simulink model "Switch"  (R2024b)
settings: Solver=VariableStepAuto  StartTime=0.0  StopTime=1  FixedStep=50e-6  MaxStep=0.001  MinStep=1e-8
model workspace (MAT data in the model file):
  condition = Simulink.Parameter
  condition.Complexity = 'real'
  condition.Dimensions = [0 0]
  condition.DataType = 'auto'
undefined symbols (not defined in the file or in its folder): DiscIntNeverNeededParam, ee_sli_rtmsupport, gcbh
libraries: spsIdealSwitchLib x12, spsCurrentMeasurementLib x6, spsSeriesRLCBranchLib x6, eeGeneralControl x6, spsControlledVoltageSourceLib x6, spsVoltageMeasurementLib x6, simulink x3, spsAsynchronousMachineSIUnitsLib x2, spsGroundLib x2, spsThreePhaseTransformerInductanceMatrixTypeTwoWindingsLib x1, spspowerguiLib x1
(part 1 of 2)
settings Model: Creator=rishikeshtiwari  LastModifiedBy=Milan Mavani
settings DebuggingCC: IgnoredZcDiagnostic=none

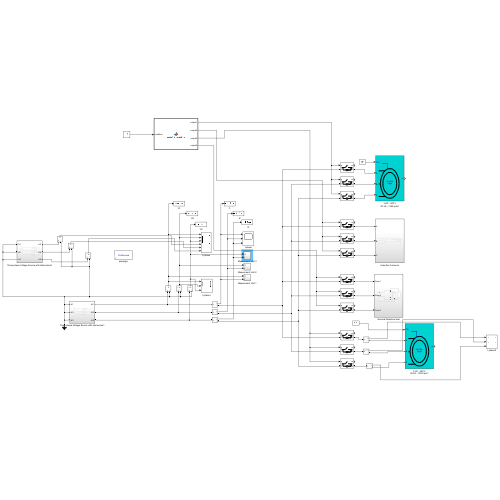
[thumbnail: Simulink's stored preview of the top-level diagram]
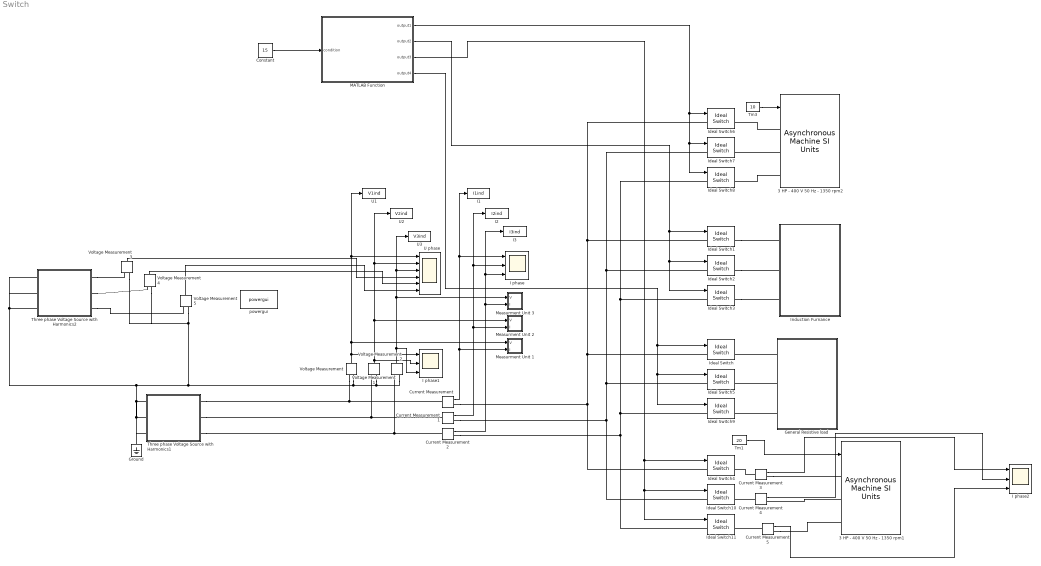
== system Switch ==
  "    I2" : ToWorkspace  VariableName=I2ind  SaveFormat=Timeseries  SampleTime=0.001
  "    I3" : ToWorkspace  VariableName=I3ind  SaveFormat=Timeseries  SampleTime=0.001
  3 HP - 400 V 50 Hz - 1350 rpm1 : spsAsynchronousMachineSIUnitsLib/Asynchronous Machine SI Units  RotorType=Double squirrel-cage  PresetModel=No  MechanicalLoad=Torque Tm  ShowDetailedParameters=on  ReferenceFrame=Stationary  Units=SI  MeasurementBus=on  NominalParameters=[2985 400 50]  VoltageRatio=1  Stator=[3.244 0.00018]  Rotor="[ 0.816  2.0e-3 ]"  Cage1=[1.701 0.01278]  Cage2=[2.063 0.00018]  Lm=0.008931  Mechanical=[0.089 0 1]  PolePairs=2  InitialConditions="[ 1,0   0,0,0   0,0,0 ]"  SimulateSaturation=off  Saturation=[14.03593122, 27.81365428, 53.79336849, 72.68890987, 97.98006896, 148.6815601, 215.7428561, 302.9841135, 428.7778367 ; 230, 322, 414, 460, 506, 552, 598, 644, 690]  LoadFlowParameters=0  TsPowergui=0  TsBlock=-1  IterativeModel=Trapezoidal non iterative  IterativeDiscreteModel=Trapezoidal non iterative  Pmec=0
      settings: AttributesFormatString=\n
  3 HP - 400 V 50 Hz - 1350 rpm2 : spsAsynchronousMachineSIUnitsLib/Asynchronous Machine SI Units  RotorType=Double squirrel-cage  PresetModel=No  MechanicalLoad=Torque Tm  ShowDetailedParameters=on  ReferenceFrame=Stationary  Units=SI  MeasurementBus=on  NominalParameters=[1720.1 400 50]  VoltageRatio=1  Stator=[76.66 0.08155]  Rotor="[ 0.816  2.0e-3 ]"  Cage1=[87.17 0.08486]  Cage2=[87.63 0.08155]  Lm=0.8867  Mechanical=[0.089 0 2]  PolePairs=2  InitialConditions="[ 1,0   0,0,0   0,0,0 ]"  SimulateSaturation=off  Saturation=[14.03593122, 27.81365428, 53.79336849, 72.68890987, 97.98006896, 148.6815601, 215.7428561, 302.9841135, 428.7778367 ; 230, 322, 414, 460, 506, 552, 598, 644, 690]  LoadFlowParameters=0  TsPowergui=0  TsBlock=-1  IterativeModel=Trapezoidal non iterative  IterativeDiscreteModel=Trapezoidal non iterative  Pmec=0
      settings: AttributesFormatString=\n
  Constant : Constant  Value=15  VectorParams1D=off  OutDataTypeStr=Inherit: Inherit via back propagation
  Current Measurement{,1..5} (6 alike) : spsCurrentMeasurementLib/Current Measurement  PhasorSimulation=off  OutputType=Complex  PSBequivalent=0
  General Resistive load : Subsystem
  Ground : spsGroundLib/Ground  LConnTagsString=a
  I phase : Scope  NumInputPorts=3
  I phase1 : Scope  NumInputPorts=3
  I phase2 : Scope  NumInputPorts=3
  I1 : ToWorkspace  VariableName=I1ind  SaveFormat=Timeseries  SampleTime=0.001
  Ideal Switch{,1..11} (12 alike) : spsIdealSwitchLib/Ideal Switch  Ron=0.001  Lon=0  IC=0  Rs=1e10  Cs=inf  Measurements=on
  Induction Furnance : Subsystem
  MATLAB Function : MATLAB Function  TreatAsAtomicUnit=on
  Measurment Unit 1 : Subsystem
  Measurment Unit 2 : Subsystem
  Measurment Unit 3 : Subsystem
  Three phase Voltage Source with Harmonics1 : Subsystem
  Three phase Voltage Source with Harmonics2 : Subsystem
  Tm1 : Constant  Value=20
  Tm3 : Constant  Value=10
  U phase : Scope  NumInputPorts=6
  U1 : ToWorkspace  VariableName=V1ind  SaveFormat=Timeseries  SampleTime=0.001
  U2 : ToWorkspace  VariableName=V2ind  SaveFormat=Timeseries  SampleTime=0.001
  U3 : ToWorkspace  VariableName=V3ind  SaveFormat=Timeseries  SampleTime=0.001
  Voltage Measurement{,1..5} (6 alike) : spsVoltageMeasurementLib/Voltage Measurement  PhasorSimulation=off  OutputType=Complex  PSBequivalent=0
  powergui : spspowerguiLib/powergui  Priority=1  SimulationMode=Continuous  SampleTime=50e-6  frequency=60  Iterations=50  frequencyindice=50  Pbase=100e6  ErrMax=1e-4  UnitsV=kV  UnitsW=MW  buscounter=0  FunctionMessages=off  echomessages=off  EnableUseOfTLC=off  CurrentSourceSwitches=off  DisableSnubberDevices=off  DisableRonSwitches=off  DisableVfSwitches=off  DisplayEquations=off  AutomaticDiscreteSolvers=off  SolverType=Tustin/Backward Euler (TBE)  Interpol=off  ExternalGateDelay=off  methode=off  Ts=100  x0status=blocks  SPID=on  SwTol=0  HookPort=off  NonlinearTolerance=1e-4  nMaxIteration=100  ContinueOnMaxIteration=off  RestoreLinks=warning  ResistiveCurrentMeasurement=off  Frange=[0:2:500]  Ylog=off  Xlog=on  ShowGrid=off  save=off  variable=ZData  structure=0  ZoomFFT=off  StartTime=0.0  cycles=1  DisplayStyle=1  fundamental=60  FreqAxis=off  MaxFrequency=1000  frequencyindicesteady=1  RmsSteady=1  display=off
  wires:
  Tm3/1 -> 3 HP - 400 V 50 Hz - 1350 rpm2/1
  Current Measurement/1 -> Measurment Unit 1/2(I), I1/1, I phase/1
  Current Measurement1/1 -> "    I2"/1, I phase/2, Measurment Unit 2/2(I)
  Current Measurement2/1 -> "    I3"/1, I phase/3, Measurment Unit 3/2(I)
  Voltage Measurement1/1 -> I phase1/2, U2/1, U phase/2, Measurment Unit 2/1(V)
  Voltage Measurement/1 -> I phase1/1, Measurment Unit 1/1(V), U1/1, U phase/1
  MATLAB Function/2(output2) -> Ideal Switch3/1, Ideal Switch2/1, Ideal Switch1/1
  Constant/1 -> MATLAB Function/1(condition)
  MATLAB Function/4(output4) -> Ideal Switch/1, Ideal Switch5/1, Ideal Switch9/1
  MATLAB Function/3(output3) -> Ideal Switch4/1, Ideal Switch10/1, Ideal Switch11/1
  Voltage Measurement3/1 -> U phase/4
  Voltage Measurement4/1 -> U phase/5
  Voltage Measurement5/1 -> U phase/6
  MATLAB Function/1(output1) -> Ideal Switch8/1, Ideal Switch7/1, Ideal Switch6/1
  Tm1/1 -> 3 HP - 400 V 50 Hz - 1350 rpm1/1
  Voltage Measurement2/1 -> U3/1, U phase/3, Measurment Unit 3/1(V), I phase1/3
  Current Measurement3/1 -> I phase2/1
  Current Measurement4/1 -> I phase2/2
  Current Measurement5/1 -> I phase2/3
  connections:
  3 HP - 400 V 50 Hz - 1350 rpm2/LConn2 -- Ideal Switch7/RConn1
  3 HP - 400 V 50 Hz - 1350 rpm2/LConn3 -- Ideal Switch8/RConn1
  3 HP - 400 V 50 Hz - 1350 rpm2/LConn1 -- Ideal Switch6/RConn1
  Voltage Measurement/LConn1 -- Three phase Voltage Source with Harmonics1/RConn1 -- Current Measurement/LConn1
  Voltage Measurement1/LConn2 -- Voltage Measurement2/LConn2 -- Three phase Voltage Source with Harmonics1/LConn1 -- Three phase Voltage Source with Harmonics1/LConn2 -- Three phase Voltage Source with Harmonics1/LConn3 -- Ground/LConn1 -- Three phase Voltage Source with Harmonics2/LConn3 -- Three phase Voltage Source with Harmonics2/LConn2 -- Three phase Voltage Source with Harmonics2/LConn1 -- Voltage Measurement3/LConn2 -- Voltage Measurement4/LConn2 -- Voltage Measurement5/LConn2 -- Voltage Measurement/LConn2
  Current Measurement2/LConn1 -- Three phase Voltage Source with Harmonics1/RConn3 -- Voltage Measurement2/LConn1
  Current Measurement1/LConn1 -- Three phase Voltage Source with Harmonics1/RConn2 -- Voltage Measurement1/LConn1
  Current Measurement/RConn1 -- Ideal Switch/LConn1 -- Ideal Switch6/LConn1 -- Ideal Switch1/LConn1 -- Ideal Switch4/LConn1
  Current Measurement1/RConn1 -- Ideal Switch2/LConn1 -- Ideal Switch7/LConn1 -- Ideal Switch5/LConn1 -- Ideal Switch10/LConn1
  Current Measurement2/RConn1 -- Ideal Switch9/LConn1 -- Ideal Switch3/LConn1 -- Ideal Switch8/LConn1 -- Ideal Switch11/LConn1
  General Resistive load/LConn1 -- Ideal Switch/RConn1
  General Resistive load/LConn2 -- Ideal Switch5/RConn1
  General Resistive load/LConn3 -- Ideal Switch9/RConn1
  Ideal Switch1/RConn1 -- Induction Furnance/LConn1
  Ideal Switch2/RConn1 -- Induction Furnance/LConn2
  Ideal Switch3/RConn1 -- Induction Furnance/LConn3
  Three phase Voltage Source with Harmonics2/RConn1 -- Voltage Measurement3/LConn1
  Three phase Voltage Source with Harmonics2/RConn2 -- Voltage Measurement4/LConn1
  Three phase Voltage Source with Harmonics2/RConn3 -- Voltage Measurement5/LConn1
  Current Measurement5/LConn1 -- Ideal Switch11/RConn1
  Current Measurement4/LConn1 -- Ideal Switch10/RConn1
  Current Measurement3/LConn1 -- Ideal Switch4/RConn1
  Current Measurement3/RConn1 -- 3 HP - 400 V 50 Hz - 1350 rpm1/LConn1
  3 HP - 400 V 50 Hz - 1350 rpm1/LConn2 -- Current Measurement4/RConn1
  Current Measurement5/RConn1 -- 3 HP - 400 V 50 Hz - 1350 rpm1/LConn3

== system Switch/General Resistive load ==
  Series RLC Branch : spsSeriesRLCBranchLib/Series RLC Branch  LConnTagsString=__new0  RConnTagsString=__new0  BranchType=R  Resistance=6.16  Inductance=0  SetiL0=off  InitialCurrent=0  Capacitance=1e-6  Setx0=off  InitialVoltage=0  Measurements=None
  Series RLC Branch1 : spsSeriesRLCBranchLib/Series RLC Branch  LConnTagsString=__new0  RConnTagsString=__new0  BranchType=R  Resistance=6.16  Inductance=0  SetiL0=off  InitialCurrent=0  Capacitance=1e-6  Setx0=off  InitialVoltage=0  Measurements=None
  Series RLC Branch2 : spsSeriesRLCBranchLib/Series RLC Branch  LConnTagsString=__new0  RConnTagsString=__new0  BranchType=R  Resistance=6.16  Inductance=0  SetiL0=off  InitialCurrent=0  Capacitance=1e-6  Setx0=off  InitialVoltage=0  Measurements=None
  Conn1 : PMIOPort  Side=Left
  Conn2 : PMIOPort  Port=2  Side=Left
  Conn3 : PMIOPort  Port=3  Side=Left
  connections:
  Series RLC Branch1/RConn1 -- Conn3/RConn1 -- Series RLC Branch2/RConn1
  Series RLC Branch/RConn1 -- Conn2/RConn1 -- Series RLC Branch1/LConn1
  Series RLC Branch/LConn1 -- Series RLC Branch2/LConn1 -- Conn1/RConn1

== system Switch/Induction Furnance ==
  Ground1 : spsGroundLib/Ground  LConnTagsString=a
  Series RL Branch : spsSeriesRLCBranchLib/Series RLC Branch  LConnTagsString=__new0  RConnTagsString=__new0  BranchType=RL  Resistance=157.6  Inductance=0.3006  SetiL0=off  InitialCurrent=0  Capacitance=1e-6  Setx0=off  InitialVoltage=0  Measurements=None
  Series RL Branch1 : spsSeriesRLCBranchLib/Series RLC Branch  LConnTagsString=__new0  RConnTagsString=__new0  BranchType=RL  Resistance=157.6  Inductance=0.3006  SetiL0=off  InitialCurrent=0  Capacitance=1e-6  Setx0=off  InitialVoltage=0  Measurements=None
  Series RL Branch2 : spsSeriesRLCBranchLib/Series RLC Branch  LConnTagsString=__new0  RConnTagsString=__new0  BranchType=RL  Resistance=157.6  Inductance=0.3006  SetiL0=off  InitialCurrent=0  Capacitance=1e-6  Setx0=off  InitialVoltage=0  Measurements=None
  Step up transformer : spsThreePhaseTransformerInductanceMatrixTypeTwoWindingsLib/Three-Phase Transformer Inductance Matrix Type (Two Windings)  CoreType=Three single-phase cores  Winding1Connection=Yg  Winding2Connection=Yg  AutoTransformer=off  Measurements=None  NominalPower=[100e3, 50]  VLLnom=[400, 3300]  WindingResistances=[0.01, 0.01]  NoLoadIexcPos=2  NoLoadPlossPos=1000  ShortCircuitReactancePos=0.06  ShortCircuitReactancePosAuto=0.06  NoLoadIexcZero=100  NoLoadPlossZero=1500  ShortCircuitReactanceZero=0.03  ShortCircuitReactanceZeroAuto=0.03
      settings: LibrarySourceBlock=|
      | sps_lib/Power Grid Elements/Three-Phase Transformer
      | Inductance Matrix Type
      | (Two Windings)
  A : PMIOPort  Side=Left
  B : PMIOPort  Port=2  Side=Left
  C : PMIOPort  Port=3  Side=Left
  connections:
  Step up transformer/RConn2 -- Series RL Branch1/RConn1
  Series RL Branch2/RConn1 -- Step up transformer/RConn3
  Series RL Branch/RConn1 -- Step up transformer/RConn1
  B/RConn1 -- Step up transformer/LConn2
  Ground1/LConn1 -- Series RL Branch/LConn1 -- Series RL Branch1/LConn1 -- Series RL Branch2/LConn1
  C/RConn1 -- Step up transformer/LConn3
  A/RConn1 -- Step up transformer/LConn1

== system Switch/Measurment Unit 1 ==
  V : Inport
  I : Inport  Port=2
  Add1 : Sum
  Divide : Product  Inputs=*/
  Math Function : Math  Operator=square
  Math Function1 : Math  Operator=square
  Power Measurement : Subsystem  AncestorBlock=ee_sl_lib/Measurements/Power Measurement  LoadFcn=ee_sli_rtmsupport( 'loadfcn', gcbh );  Variant=on  VariantControlMode=label  LabelModeActiveChoice=Continuous  mask(Power Measurement){F=50, K=[1 3 5 7], Ts=0}
      mask prompts: F "physmod:ee:library:comments:control:eePowerMeasurement:BaseFrequencyHz_MP"; K "physmod:ee:library:comments:control:eePowerMeasurement:HarmonicNumbers_MP"; Ts "physmod:ee:library:comments:control:eePowerMeasurement:SampleTime_MP"
      mask help: physmod:ee:library:comments:control:eePowerMeasurement:PowerMeasurement_MD
      mask init:
      | timeDomain=ee.mask.initializePowerMeasurement(gcb,F,Ts);
      settings: CopyFcn=ee_sli_rtmsupport( 'copyfcn', gcbh );  DeleteFcn=ee_sli_rtmsupport( 'deletefcn', gcbh );  ModelCloseFcn=ee_sli_rtmsupport( 'modelclosefcn', gcbh );  PostSaveFcn=ee_sli_rtmsupport( 'postsavefcn', gcbh );  PreCopyFcn=ee_sli_rtmsupport( 'precopyfcn', gcbh );  OpenFcn=ee_sli_rtmsupport( 'openfcn', gcbh );  CloseFcn=ee_sli_rtmsupport( 'closefcn', gcbh );  PreDeleteFcn=ee_sli_rtmsupport( 'predeletefcn', gcbh );
      settings: LibrarySourceBlock=|
      | ee_sl_lib/Measurements/Power
      | Measurement
      mask Help: web(nesl_help(gcbh))
      mask Display: ee.mask.drawPowerMeasurement();
  Sqrt : Sqrt
  To Workspace6 : ToWorkspace  VariableName=P1  SaveFormat=Timeseries  SampleTime=0.001
  To Workspace7 : ToWorkspace  VariableName=Q1  SaveFormat=Timeseries  SampleTime=0.001
  To Workspace8 : ToWorkspace  VariableName=A1  SaveFormat=Timeseries  SampleTime=0.001
  wires:
  Math Function1/1 -> Add1/2
  Power Measurement/2(Q) -> To Workspace7/1, Math Function1/1
  Add1/1 -> Sqrt/1
  Sqrt/1 -> To Workspace8/1, Divide/2
  Power Measurement/1(P) -> To Workspace6/1, Divide/1, Math Function/1
  Math Function/1 -> Add1/1
  V/1 -> Power Measurement/1(v)
  I/1 -> Power Measurement/2(i)

== system Switch/Measurment Unit 2 ==
  V : Inport
  I : Inport  Port=2
  Add2 : Sum
  Math Function2 : Math  Operator=square
  Math Function3 : Math  Operator=square
  Power Measurement : Subsystem  AncestorBlock=ee_sl_lib/Measurements/Power Measurement  LoadFcn=ee_sli_rtmsupport( 'loadfcn', gcbh );  Variant=on  VariantControlMode=label  LabelModeActiveChoice=Continuous  mask(Power Measurement){F=50, K=[1 3 5 7], Ts=0}
      mask prompts: F "physmod:ee:library:comments:control:eePowerMeasurement:BaseFrequencyHz_MP"; K "physmod:ee:library:comments:control:eePowerMeasurement:HarmonicNumbers_MP"; Ts "physmod:ee:library:comments:control:eePowerMeasurement:SampleTime_MP"
      mask help: physmod:ee:library:comments:control:eePowerMeasurement:PowerMeasurement_MD
      mask init:
      | timeDomain=ee.mask.initializePowerMeasurement(gcb,F,Ts);
      settings: CopyFcn=ee_sli_rtmsupport( 'copyfcn', gcbh );  DeleteFcn=ee_sli_rtmsupport( 'deletefcn', gcbh );  ModelCloseFcn=ee_sli_rtmsupport( 'modelclosefcn', gcbh );  PostSaveFcn=ee_sli_rtmsupport( 'postsavefcn', gcbh );  PreCopyFcn=ee_sli_rtmsupport( 'precopyfcn', gcbh );  OpenFcn=ee_sli_rtmsupport( 'openfcn', gcbh );  CloseFcn=ee_sli_rtmsupport( 'closefcn', gcbh );  PreDeleteFcn=ee_sli_rtmsupport( 'predeletefcn', gcbh );
      settings: LibrarySourceBlock=|
      | ee_sl_lib/Measurements/Power
      | Measurement
      mask Help: web(nesl_help(gcbh))
      mask Display: ee.mask.drawPowerMeasurement();
  Sqrt1 : Sqrt
  To Workspace10 : ToWorkspace  VariableName=P2  SaveFormat=Timeseries  SampleTime=0.001
  To Workspace11 : ToWorkspace  VariableName=Q2  SaveFormat=Timeseries  SampleTime=0.001
  To Workspace12 : ToWorkspace  VariableName=A2  SaveFormat=Timeseries  SampleTime=0.001
  wires:
  Power Measurement/1(P) -> Math Function2/1, To Workspace10/1
  Math Function3/1 -> Add2/2
  Math Function2/1 -> Add2/1
  Add2/1 -> Sqrt1/1
  I/1 -> Power Measurement/2(i)
  Sqrt1/1 -> To Workspace12/1
  Power Measurement/2(Q) -> Math Function3/1, To Workspace11/1
  V/1 -> Power Measurement/1(v)

== system Switch/Measurment Unit 3 ==
  V : Inport
  I : Inport  Port=2
  Add3 : Sum
  Math Function4 : Math  Operator=square
  Math Function5 : Math  Operator=square
  Power Measurement : Subsystem  AncestorBlock=ee_sl_lib/Measurements/Power Measurement  LoadFcn=ee_sli_rtmsupport( 'loadfcn', gcbh );  Variant=on  VariantControlMode=label  LabelModeActiveChoice=Continuous  mask(Power Measurement){F=50, K=[1 3 5 7], Ts=0}
      mask prompts: F "physmod:ee:library:comments:control:eePowerMeasurement:BaseFrequencyHz_MP"; K "physmod:ee:library:comments:control:eePowerMeasurement:HarmonicNumbers_MP"; Ts "physmod:ee:library:comments:control:eePowerMeasurement:SampleTime_MP"
      mask help: physmod:ee:library:comments:control:eePowerMeasurement:PowerMeasurement_MD
      mask init:
      | timeDomain=ee.mask.initializePowerMeasurement(gcb,F,Ts);
      settings: CopyFcn=ee_sli_rtmsupport( 'copyfcn', gcbh );  DeleteFcn=ee_sli_rtmsupport( 'deletefcn', gcbh );  ModelCloseFcn=ee_sli_rtmsupport( 'modelclosefcn', gcbh );  PostSaveFcn=ee_sli_rtmsupport( 'postsavefcn', gcbh );  PreCopyFcn=ee_sli_rtmsupport( 'precopyfcn', gcbh );  OpenFcn=ee_sli_rtmsupport( 'openfcn', gcbh );  CloseFcn=ee_sli_rtmsupport( 'closefcn', gcbh );  PreDeleteFcn=ee_sli_rtmsupport( 'predeletefcn', gcbh );
      settings: LibrarySourceBlock=|
      | ee_sl_lib/Measurements/Power
      | Measurement
      mask Help: web(nesl_help(gcbh))
      mask Display: ee.mask.drawPowerMeasurement();
  Scope : Scope
  Sqrt2 : Sqrt
  To Workspace14 : ToWorkspace  VariableName=P3  SaveFormat=Timeseries  SampleTime=0.001
  To Workspace15 : ToWorkspace  VariableName=Q3  SaveFormat=Timeseries  SampleTime=0.001
  To Workspace16 : ToWorkspace  VariableName=A3  SaveFormat=Timeseries  SampleTime=0.001
  wires:
  Math Function5/1 -> Add3/2
  Power Measurement/1(P) -> Scope/1, Math Function4/1, To Workspace14/1
  Sqrt2/1 -> To Workspace16/1
  Power Measurement/2(Q) -> Math Function5/1, To Workspace15/1
  Add3/1 -> Sqrt2/1
  V/1 -> Power Measurement/1(v)
  Math Function4/1 -> Add3/1
  I/1 -> Power Measurement/2(i)

== system Switch/Three phase Voltage Source with Harmonics1 ==
  note: Phase 1
  note: Phase 3
  note: Phase 2
  "  " : spsControlledVoltageSourceLib/Controlled Voltage Source  Initialize=on  Source_Type=AC  Amplitude=230*sqrt(2)  Phase=0  Frequency=50  Measurements=None
  Controlled Voltage Source1 : spsControlledVoltageSourceLib/Controlled Voltage Source  Initialize=on  Source_Type=AC  Amplitude=230*sqrt(2)  Phase=120  Frequency=50  Measurements=None
  Controlled Voltage Source2 : spsControlledVoltageSourceLib/Controlled Voltage Source  Initialize=on  Source_Type=AC  Amplitude=230*sqrt(2)  Phase=240  Frequency=50  Measurements=None
  Harmonic phase 1 : Subsystem
  Harmonic phase 2 : Subsystem
  Harmonic phase 3 : Subsystem
  -U1 : PMIOPort  Side=Left
  -U2 : PMIOPort  Port=2  Side=Left
  -U3 : PMIOPort  Port=3  Side=Left
  +U1 : PMIOPort  Port=4  Side=Right
  +U2 : PMIOPort  Port=5  Side=Right
  +U3 : PMIOPort  Port=6  Side=Right
  wires:
  Harmonic phase 3/1(Out1) -> Controlled Voltage Source2/1
  Harmonic phase 2/1(Out1) -> Controlled Voltage Source1/1
  Harmonic phase 1/1(Out1) -> "  "/1
  connections:
  Controlled Voltage Source1/LConn1 -- -U2/RConn1
  Controlled Voltage Source2/RConn1 -- +U3/RConn1
  Controlled Voltage Source2/LConn1 -- -U3/RConn1
  "  "/RConn1 -- +U1/RConn1
  Controlled Voltage Source1/RConn1 -- +U2/RConn1
  "  "/LConn1 -- -U1/RConn1

== system Switch/Three phase Voltage Source with Harmonics2 ==
  note: Phase 2
  note: Phase 3
  note: Phase 1
  "  " : spsControlledVoltageSourceLib/Controlled Voltage Source  Initialize=on  Source_Type=AC  Amplitude=230*sqrt(2)  Phase=0  Frequency=50  Measurements=None
  Controlled Voltage Source1 : spsControlledVoltageSourceLib/Controlled Voltage Source  Initialize=on  Source_Type=AC  Amplitude=230*sqrt(2)  Phase=120  Frequency=50  Measurements=None
  Controlled Voltage Source2 : spsControlledVoltageSourceLib/Controlled Voltage Source  Initialize=on  Source_Type=AC  Amplitude=230*sqrt(2)  Phase=240  Frequency=50  Measurements=None
  Harmonic phase 1 : Subsystem
  Harmonic phase 2 : Subsystem
  Harmonic phase 3 : Subsystem
  -U1 : PMIOPort  Side=Left
  -U2 : PMIOPort  Port=2  Side=Left
  -U3 : PMIOPort  Port=3  Side=Left
  +U1 : PMIOPort  Port=4  Side=Right
  +U2 : PMIOPort  Port=5  Side=Right
  +U3 : PMIOPort  Port=6  Side=Right
  wires:
  Harmonic phase 1/1(Out1) -> "  "/1
  Harmonic phase 2/1(Out1) -> Controlled Voltage Source1/1
  Harmonic phase 3/1(Out1) -> Controlled Voltage Source2/1
  connections:
  "  "/LConn1 -- -U1/RConn1
  Controlled Voltage Source1/RConn1 -- +U2/RConn1
  "  "/RConn1 -- +U1/RConn1
  Controlled Voltage Source2/LConn1 -- -U3/RConn1
  Controlled Voltage Source2/RConn1 -- +U3/RConn1
  Controlled Voltage Source1/LConn1 -- -U2/RConn1

== system Switch/Measurment Unit 1/Power Measurement ==
  v : Inport
  i : Inport  Port=2
  Continuous : Subsystem  VariantControl=Continuous  mask(Single-phase power measurement){F=F, K=K}
      mask prompts: F "Base frequency (Hz):"; K "Harmonic numbers:"
      mask init:
      | % For an AC component, the gain is 1/2;
      | % for a DC component, the gain is 1/4.
      | 
      | G = 0.5*ones(1,length(K));
      | if ~isempty(find(K==0, 1))
      |     G(K==0) = 0.25;   
      | end
  Discrete : Subsystem  VariantControl=Discrete  mask(Single-phase power measurement){F=F, K=K, Ts=Ts}
      mask prompts: F "Base frequency (Hz):"; K "Harmonic numbers:"; Ts "Sample time (s):"
      mask init:
      | % For an AC component, the gain is 1/2;
      | % for a DC component, the gain is 1/4.
      | 
      | G = 0.5*ones(1,length(K));
      | if ~isempty(find(K==0, 1))
      |     G(K==0) = 0.25;   
      | end
  P : Outport  VectorParamsAs1DForOutWhenUnconnected=off
  Q : Outport  Port=2  VectorParamsAs1DForOutWhenUnconnected=off

== system Switch/Measurment Unit 2/Power Measurement ==
  v : Inport
  i : Inport  Port=2
  Continuous : Subsystem  VariantControl=Continuous  mask(Single-phase power measurement){F=F, K=K}
      mask prompts: F "Base frequency (Hz):"; K "Harmonic numbers:"
      mask init:
      | % For an AC component, the gain is 1/2;
      | % for a DC component, the gain is 1/4.
      | 
      | G = 0.5*ones(1,length(K));
      | if ~isempty(find(K==0, 1))
      |     G(K==0) = 0.25;   
      | end
  Discrete : Subsystem  VariantControl=Discrete  mask(Single-phase power measurement){F=F, K=K, Ts=Ts}
      mask prompts: F "Base frequency (Hz):"; K "Harmonic numbers:"; Ts "Sample time (s):"
      mask init:
      | % For an AC component, the gain is 1/2;
      | % for a DC component, the gain is 1/4.
      | 
      | G = 0.5*ones(1,length(K));
      | if ~isempty(find(K==0, 1))
      |     G(K==0) = 0.25;   
      | end
  P : Outport  VectorParamsAs1DForOutWhenUnconnected=off
  Q : Outport  Port=2  VectorParamsAs1DForOutWhenUnconnected=off

== system Switch/Measurment Unit 3/Power Measurement ==
  v : Inport
  i : Inport  Port=2
  Continuous : Subsystem  VariantControl=Continuous  mask(Single-phase power measurement){F=F, K=K}
      mask prompts: F "Base frequency (Hz):"; K "Harmonic numbers:"
      mask init:
      | % For an AC component, the gain is 1/2;
      | % for a DC component, the gain is 1/4.
      | 
      | G = 0.5*ones(1,length(K));
      | if ~isempty(find(K==0, 1))
      |     G(K==0) = 0.25;   
      | end
  Discrete : Subsystem  VariantControl=Discrete  mask(Single-phase power measurement){F=F, K=K, Ts=Ts}
      mask prompts: F "Base frequency (Hz):"; K "Harmonic numbers:"; Ts "Sample time (s):"
      mask init:
      | % For an AC component, the gain is 1/2;
      | % for a DC component, the gain is 1/4.
      | 
      | G = 0.5*ones(1,length(K));
      | if ~isempty(find(K==0, 1))
      |     G(K==0) = 0.25;   
      | end
  P : Outport  VectorParamsAs1DForOutWhenUnconnected=off
  Q : Outport  Port=2  VectorParamsAs1DForOutWhenUnconnected=off

== system Switch/Three phase Voltage Source with Harmonics1/Harmonic phase 1 ==
  3rd Harmonic : Sin  Amplitude=(230*1.4142)*0.20  Frequency=2*pi*50*3  SampleTime=50e-6
  5th Harmonic : Sin  Amplitude=(230*1.4142)*0.05  Frequency=2*pi*50*5  SampleTime=50e-6
  7th harmonic : Sin  Amplitude=(230*1.4142)*0.01  Frequency=2*pi*50*7  SampleTime=50e-6
  Add : Sum  Inputs=++++
  Fundamental : Sin  Amplitude=230*1.4142  Frequency=50*pi*2  SampleTime=50e-6
  Out1 : Outport
  wires:
  3rd Harmonic/1 -> Add/2
  7th harmonic/1 -> Add/4
  5th Harmonic/1 -> Add/3
  Add/1 -> Out1/1
  Fundamental/1 -> Add/1

== system Switch/Three phase Voltage Source with Harmonics1/Harmonic phase 2 ==
  3rd Harmonic : Sin  Amplitude=(230*1.4142)*0.20  Frequency=2*pi*50*3  SampleTime=50e-6
  5th Harmonic : Sin  Amplitude=(230*1.4142)*0.05  Frequency=2*pi*50*5  Phase=240*(pi/180)  SampleTime=50e-6
  7th Harmonic : Sin  Amplitude=(230*1.4142)*0.01  Frequency=2*pi*50*7  Phase=120*(pi/180)  SampleTime=50e-6
  Add : Sum  Inputs=++++
  Fundamental : Sin  Amplitude=230*1.4142  Frequency=50*pi*2  Phase=120*(pi/180)  SampleTime=50e-6
  Out1 : Outport
  wires:
  3rd Harmonic/1 -> Add/2
  7th Harmonic/1 -> Add/4
  5th Harmonic/1 -> Add/3
  Fundamental/1 -> Add/1
  Add/1 -> Out1/1

== system Switch/Three phase Voltage Source with Harmonics1/Harmonic phase 3 ==
  3rd Harmonic : Sin  Amplitude=(230*1.4142)*0.20  Frequency=2*pi*50*3  SampleTime=50e-6
  5th Harmonic : Sin  Amplitude=(230*1.4142)*0.05  Frequency=50*3.14*2*5  Phase=120*(pi/180)  SampleTime=50e-6
  7th Harmonic : Sin  Amplitude=(230*1.4142)*0.01  Frequency=50*3.14*2*7  Phase=240*(pi/180)  SampleTime=50e-6
  Add : Sum  Inputs=++++
  Fundamental : Sin  Amplitude=230*1.4142  Frequency=50*2*pi  Phase=240*(pi/180)  SampleTime=50e-6
  Out1 : Outport
  wires:
  7th Harmonic/1 -> Add/4
  5th Harmonic/1 -> Add/3
  Add/1 -> Out1/1
  Fundamental/1 -> Add/1
  3rd Harmonic/1 -> Add/2

== system Switch/Three phase Voltage Source with Harmonics2/Harmonic phase 1 ==
  Add : Sum  Inputs=++++
  Fundamental : Sin  Amplitude=230*1.4142  Frequency=50*pi*2  SampleTime=50e-6
  Out1 : Outport
  wires:
  Fundamental/1 -> Add/1
  Add/1 -> Out1/1

== system Switch/Three phase Voltage Source with Harmonics2/Harmonic phase 2 ==
  Add : Sum  Inputs=++++
  Fundamental : Sin  Amplitude=230*1.4142  Frequency=50*pi*2  Phase=120*(pi/180)  SampleTime=50e-6
  Out1 : Outport
  wires:
  Add/1 -> Out1/1
  Fundamental/1 -> Add/1

== system Switch/Three phase Voltage Source with Harmonics2/Harmonic phase 3 ==
  Add : Sum  Inputs=++++
  Fundamental : Sin  Amplitude=230*1.4142  Frequency=50*2*pi  Phase=240*(pi/180)  SampleTime=50e-6
  Out1 : Outport
  wires:
  Fundamental/1 -> Add/1
  Add/1 -> Out1/1

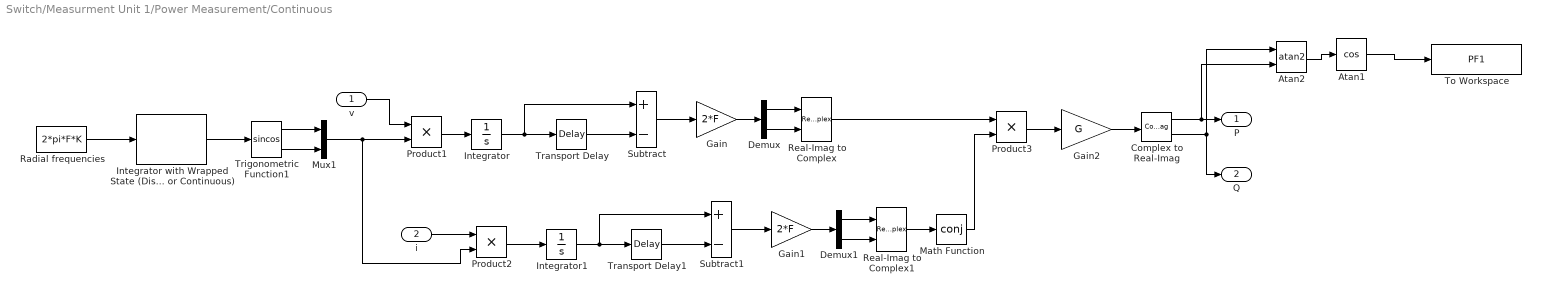
== system Switch/Measurment Unit 1/Power Measurement/Continuous ==
  v : Inport
  i : Inport  Port=2
  Atan1 : Trigonometry  Operator=cos
  Atan2 : Trigonometry  Operator=atan2
  Complex to Real-Imag : ComplexToRealImag
  Demux : Demux  Outputs=2
  Demux1 : Demux  Outputs=2
  Gain : Gain  Gain=2*F
  Gain1 : Gain  Gain=2*F
  Gain2 : Gain  Gain=G
  Integrator : Integrator
  Integrator with Wrapped State (Discrete or Continuous) : eeGeneralControl/Integrator with Wrapped State (Discrete or Continuous)  LabelModeActiveChoice=Continuous  WrappedStateUpperValue=2*pi  WrappedStateLowerValue=0  x0=0  Ts=0
  Integrator1 : Integrator
  Math Function : Math  Operator=conj  SignedPower=on
  Mux1 : Mux  Inputs=2
  Product1 : Product
  Product2 : Product
  Product3 : Product
  Radial frequencies : Constant  Value=2*pi*F*K
  Real-Imag to Complex : RealImagToComplex
  Real-Imag to Complex1 : RealImagToComplex
  Subtract : Sum  Inputs=+-
  Subtract1 : Sum  Inputs=+-
  To Workspace : ToWorkspace  VariableName=PF1  SaveFormat=Timeseries  SampleTime=0.001
  Transport Delay : TransportDelay  DelayTime=1/F  BufferSize=4096
  Transport Delay1 : TransportDelay  DelayTime=1/F  BufferSize=4096
  Trigonometric Function1 : Trigonometry  Operator=sincos
  P : Outport  VectorParamsAs1DForOutWhenUnconnected=off
  Q : Outport  Port=2  VectorParamsAs1DForOutWhenUnconnected=off
  wires:
  Integrator1/1 -> Subtract1/1, Transport Delay1/1
  Transport Delay1/1 -> Subtract1/2
  Subtract1/1 -> Gain1/1
  Demux1/1 -> Real-Imag to Complex1/1
  Gain1/1 -> Demux1/1
  Demux1/2 -> Real-Imag to Complex1/2
  Product2/1 -> Integrator1/1
  Mux1/1 -> Product1/2, Product2/2
  v/1 -> Product1/1
  Product1/1 -> Integrator/1
  Trigonometric Function1/1 -> Mux1/1
  Demux/2 -> Real-Imag to Complex/2
  Gain/1 -> Demux/1
  Demux/1 -> Real-Imag to Complex/1
  Gain2/1 -> Complex to Real-Imag/1
  Real-Imag to Complex1/1 -> Math Function/1
  Integrator with Wrapped State (Discrete or Continuous)/1 -> Trigonometric Function1/1
  Complex to Real-Imag/2 -> Q/1, Atan2/1
  Complex to Real-Imag/1 -> Atan2/2, P/1
  Real-Imag to Complex/1 -> Product3/1
  Product3/1 -> Gain2/1
  Math Function/1 -> Product3/2
  i/1 -> Product2/1
  Subtract/1 -> Gain/1
  Transport Delay/1 -> Subtract/2
  Integrator/1 -> Transport Delay/1, Subtract/1
  Radial frequencies/1 -> Integrator with Wrapped State (Discrete or Continuous)/1
  Trigonometric Function1/2 -> Mux1/2
  Atan2/1 -> Atan1/1
  Atan1/1 -> To Workspace/1

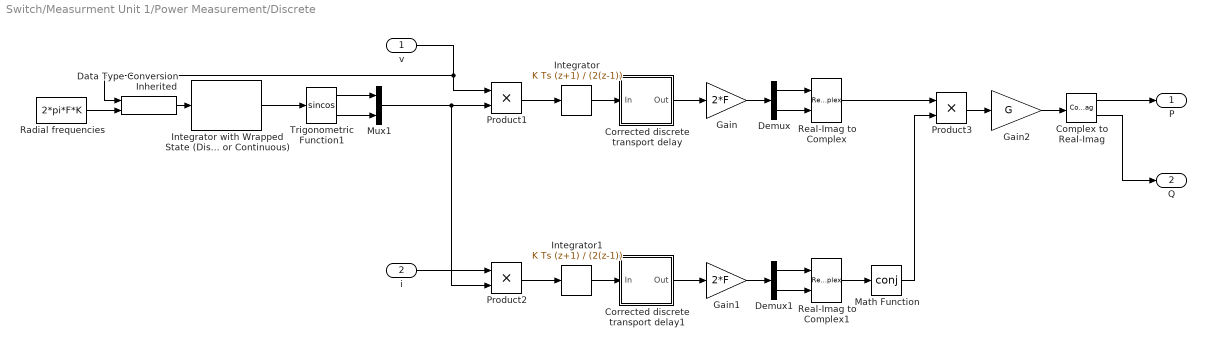
== system Switch/Measurment Unit 1/Power Measurement/Discrete ==
  v : Inport
  i : Inport  Port=2
  Complex to Real-Imag : ComplexToRealImag
  Corrected discrete transport delay : Subsystem
  Corrected discrete transport delay1 : Subsystem
  Data Type Conversion Inherited : simulink/Signal Attributes/Data Type Conversion Inherited  ConvertRealWorld=Real World Value  DoSatur=off
  Demux : Demux  Outputs=2
  Demux1 : Demux  Outputs=2
  Gain : Gain  Gain=2*F
  Gain1 : Gain  Gain=2*F
  Gain2 : Gain  Gain=G
  Integrator : DiscreteIntegrator  IntegratorMethod=Integration: Trapezoidal  SampleTime=Ts  ICPrevOutput=DiscIntNeverNeededParam  ICPrevScaledInput=DiscIntNeverNeededParam  mask(DiscretizedDiscreteIntegrator){}
      mask init:
      | %zoh
  Integrator with Wrapped State (Discrete or Continuous) : eeGeneralControl/Integrator with Wrapped State (Discrete or Continuous)  LabelModeActiveChoice=Continuous  WrappedStateUpperValue=2*pi  WrappedStateLowerValue=0  x0=0  Ts=Ts
  Integrator1 : DiscreteIntegrator  IntegratorMethod=Integration: Trapezoidal  SampleTime=Ts  ICPrevOutput=DiscIntNeverNeededParam  ICPrevScaledInput=DiscIntNeverNeededParam  mask(DiscretizedDiscreteIntegrator){}
      mask init:
      | %zoh
  Math Function : Math  Operator=conj  SignedPower=on
  Mux1 : Mux  Inputs=2
  Product1 : Product
  Product2 : Product
  Product3 : Product
  Radial frequencies : Constant  Value=2*pi*F*K
  Real-Imag to Complex : RealImagToComplex
  Real-Imag to Complex1 : RealImagToComplex
  Trigonometric Function1 : Trigonometry  Operator=sincos
  P : Outport  VectorParamsAs1DForOutWhenUnconnected=off
  Q : Outport  Port=2  VectorParamsAs1DForOutWhenUnconnected=off
  wires:
  Product2/1 -> Integrator1/1
  Demux/1 -> Real-Imag to Complex/1
  Demux1/2 -> Real-Imag to Complex1/2
  Real-Imag to Complex/1 -> Product3/1
  Complex to Real-Imag/1 -> P/1
  Real-Imag to Complex1/1 -> Math Function/1
  Corrected discrete transport delay1/1(Out) -> Gain1/1
  Demux/2 -> Real-Imag to Complex/2
  Integrator with Wrapped State (Discrete or Continuous)/1 -> Trigonometric Function1/1
  Math Function/1 -> Product3/2
  Corrected discrete transport delay/1(Out) -> Gain/1
  Trigonometric Function1/1 -> Mux1/1
  Gain/1 -> Demux/1
  Complex to Real-Imag/2 -> Q/1
  i/1 -> Product2/1
  Integrator1/1 -> Corrected discrete transport delay1/1(In)
  v/1 -> Data Type Conversion Inherited/1, Product1/1
  Gain1/1 -> Demux1/1
  Product1/1 -> Integrator/1
  Product3/1 -> Gain2/1
  Demux1/1 -> Real-Imag to Complex1/1
  Gain2/1 -> Complex to Real-Imag/1
  Integrator/1 -> Corrected discrete transport delay/1(In)
  Mux1/1 -> Product1/2, Product2/2
  Trigonometric Function1/2 -> Mux1/2
  Data Type Conversion Inherited/1 -> Integrator with Wrapped State (Discrete or Continuous)/1
  Radial frequencies/1 -> Data Type Conversion Inherited/2

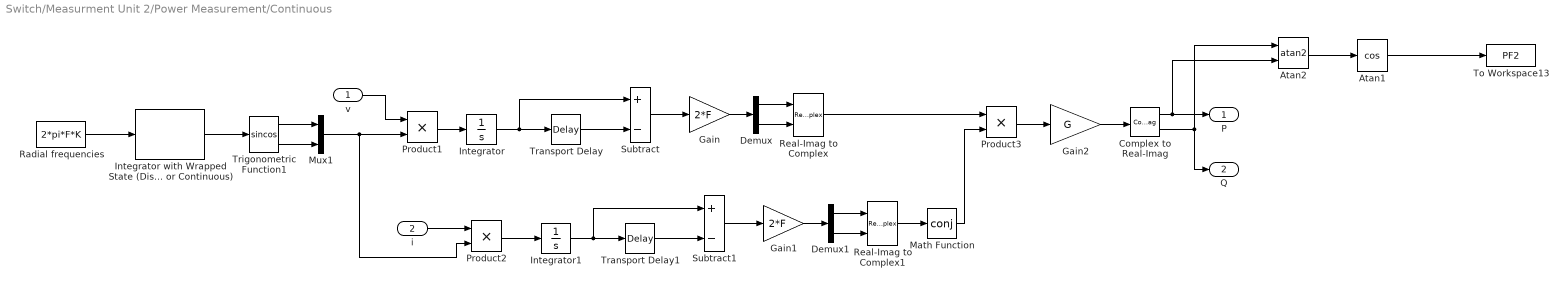
== system Switch/Measurment Unit 2/Power Measurement/Continuous ==
  v : Inport
  i : Inport  Port=2
  Atan1 : Trigonometry  Operator=cos
  Atan2 : Trigonometry  Operator=atan2
  Complex to Real-Imag : ComplexToRealImag
  Demux : Demux  Outputs=2
  Demux1 : Demux  Outputs=2
  Gain : Gain  Gain=2*F
  Gain1 : Gain  Gain=2*F
  Gain2 : Gain  Gain=G
  Integrator : Integrator
  Integrator with Wrapped State (Discrete or Continuous) : eeGeneralControl/Integrator with Wrapped State (Discrete or Continuous)  LabelModeActiveChoice=Continuous  WrappedStateUpperValue=2*pi  WrappedStateLowerValue=0  x0=0  Ts=0
  Integrator1 : Integrator
  Math Function : Math  Operator=conj  SignedPower=on
  Mux1 : Mux  Inputs=2
  Product1 : Product
  Product2 : Product
  Product3 : Product
  Radial frequencies : Constant  Value=2*pi*F*K
  Real-Imag to Complex : RealImagToComplex
  Real-Imag to Complex1 : RealImagToComplex
  Subtract : Sum  Inputs=+-
  Subtract1 : Sum  Inputs=+-
  To Workspace13 : ToWorkspace  VariableName=PF2  SaveFormat=Timeseries  SampleTime=0.001
  Transport Delay : TransportDelay  DelayTime=1/F  BufferSize=4096
  Transport Delay1 : TransportDelay  DelayTime=1/F  BufferSize=4096
  Trigonometric Function1 : Trigonometry  Operator=sincos
  P : Outport  VectorParamsAs1DForOutWhenUnconnected=off
  Q : Outport  Port=2  VectorParamsAs1DForOutWhenUnconnected=off
  wires:
  Trigonometric Function1/2 -> Mux1/2
  Radial frequencies/1 -> Integrator with Wrapped State (Discrete or Continuous)/1
  Integrator/1 -> Subtract/1, Transport Delay/1
  Transport Delay/1 -> Subtract/2
  Subtract/1 -> Gain/1
  i/1 -> Product2/1
  Math Function/1 -> Product3/2
  Product3/1 -> Gain2/1
  Real-Imag to Complex/1 -> Product3/1
  Complex to Real-Imag/1 -> Atan2/2, P/1
  Complex to Real-Imag/2 -> Q/1, Atan2/1
  Integrator with Wrapped State (Discrete or Continuous)/1 -> Trigonometric Function1/1
  Real-Imag to Complex1/1 -> Math Function/1
  Gain2/1 -> Complex to Real-Imag/1
  Demux/1 -> Real-Imag to Complex/1
  Gain/1 -> Demux/1
  Demux/2 -> Real-Imag to Complex/2
  Trigonometric Function1/1 -> Mux1/1
  Product1/1 -> Integrator/1
  v/1 -> Product1/1
  Mux1/1 -> Product2/2, Product1/2
  Product2/1 -> Integrator1/1
  Demux1/2 -> Real-Imag to Complex1/2
  Gain1/1 -> Demux1/1
  Demux1/1 -> Real-Imag to Complex1/1
  Subtract1/1 -> Gain1/1
  Transport Delay1/1 -> Subtract1/2
  Integrator1/1 -> Transport Delay1/1, Subtract1/1
  Atan2/1 -> Atan1/1
  Atan1/1 -> To Workspace13/1

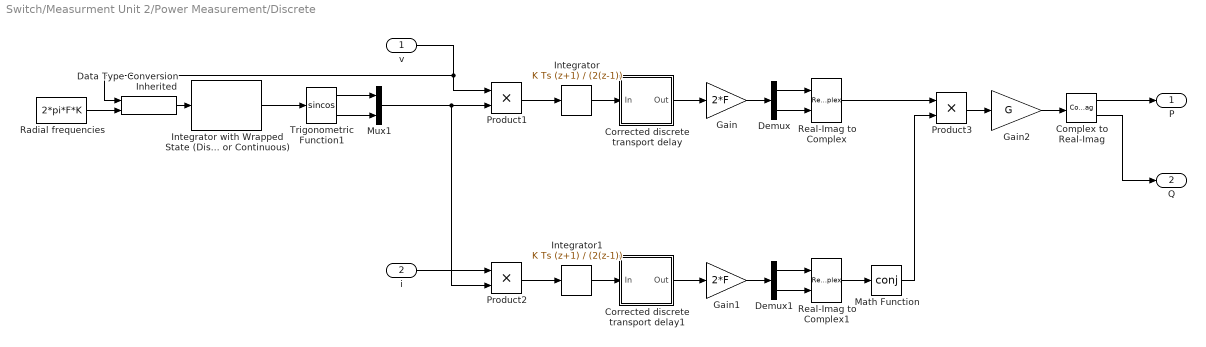
== system Switch/Measurment Unit 2/Power Measurement/Discrete ==
  v : Inport
  i : Inport  Port=2
  Complex to Real-Imag : ComplexToRealImag
  Corrected discrete transport delay : Subsystem
  Corrected discrete transport delay1 : Subsystem
  Data Type Conversion Inherited : simulink/Signal Attributes/Data Type Conversion Inherited  ConvertRealWorld=Real World Value  DoSatur=off
  Demux : Demux  Outputs=2
  Demux1 : Demux  Outputs=2
  Gain : Gain  Gain=2*F
  Gain1 : Gain  Gain=2*F
  Gain2 : Gain  Gain=G
  Integrator : DiscreteIntegrator  IntegratorMethod=Integration: Trapezoidal  SampleTime=Ts  ICPrevOutput=DiscIntNeverNeededParam  ICPrevScaledInput=DiscIntNeverNeededParam  mask(DiscretizedDiscreteIntegrator){}
      mask init:
      | %zoh
  Integrator with Wrapped State (Discrete or Continuous) : eeGeneralControl/Integrator with Wrapped State (Discrete or Continuous)  LabelModeActiveChoice=Continuous  WrappedStateUpperValue=2*pi  WrappedStateLowerValue=0  x0=0  Ts=Ts
  Integrator1 : DiscreteIntegrator  IntegratorMethod=Integration: Trapezoidal  SampleTime=Ts  ICPrevOutput=DiscIntNeverNeededParam  ICPrevScaledInput=DiscIntNeverNeededParam  mask(DiscretizedDiscreteIntegrator){}
      mask init:
      | %zoh
  Math Function : Math  Operator=conj  SignedPower=on
  Mux1 : Mux  Inputs=2
  Product1 : Product
  Product2 : Product
  Product3 : Product
  Radial frequencies : Constant  Value=2*pi*F*K
  Real-Imag to Complex : RealImagToComplex
  Real-Imag to Complex1 : RealImagToComplex
  Trigonometric Function1 : Trigonometry  Operator=sincos
  P : Outport  VectorParamsAs1DForOutWhenUnconnected=off
  Q : Outport  Port=2  VectorParamsAs1DForOutWhenUnconnected=off
  wires:
  Radial frequencies/1 -> Data Type Conversion Inherited/2
  Data Type Conversion Inherited/1 -> Integrator with Wrapped State (Discrete or Continuous)/1
  Trigonometric Function1/2 -> Mux1/2
  Mux1/1 -> Product2/2, Product1/2
  Integrator/1 -> Corrected discrete transport delay/1(In)
  Gain2/1 -> Complex to Real-Imag/1
  Demux1/1 -> Real-Imag to Complex1/1
  Product3/1 -> Gain2/1
  Product1/1 -> Integrator/1
  Gain1/1 -> Demux1/1
  v/1 -> Product1/1, Data Type Conversion Inherited/1
  Integrator1/1 -> Corrected discrete transport delay1/1(In)
  i/1 -> Product2/1
  Complex to Real-Imag/2 -> Q/1
  Gain/1 -> Demux/1
  Trigonometric Function1/1 -> Mux1/1
  Corrected discrete transport delay/1(Out) -> Gain/1
  Math Function/1 -> Product3/2
  Integrator with Wrapped State (Discrete or Continuous)/1 -> Trigonometric Function1/1
  Demux/2 -> Real-Imag to Complex/2
  Corrected discrete transport delay1/1(Out) -> Gain1/1
  Real-Imag to Complex1/1 -> Math Function/1
  Complex to Real-Imag/1 -> P/1
  Real-Imag to Complex/1 -> Product3/1
  Demux1/2 -> Real-Imag to Complex1/2
  Demux/1 -> Real-Imag to Complex/1
  Product2/1 -> Integrator1/1

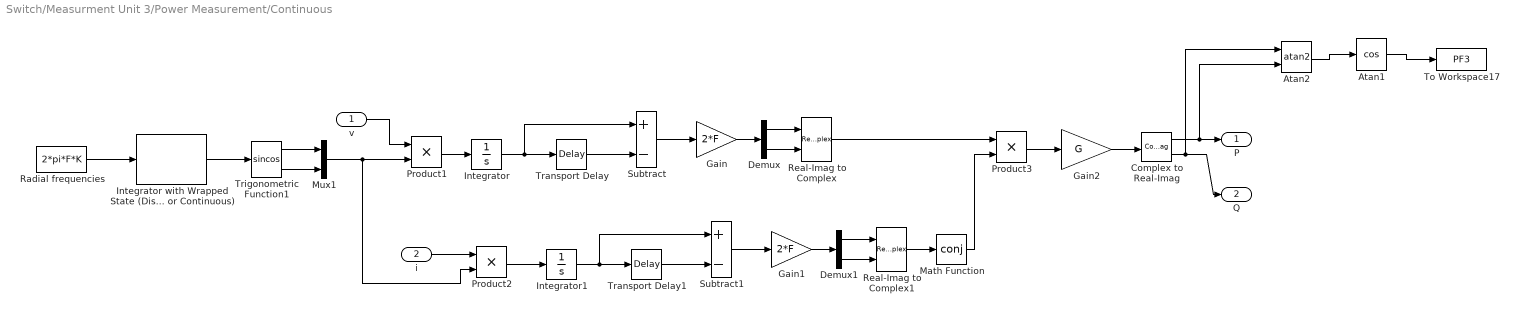
== system Switch/Measurment Unit 3/Power Measurement/Continuous ==
  v : Inport
  i : Inport  Port=2
  Atan1 : Trigonometry  Operator=cos
  Atan2 : Trigonometry  Operator=atan2
  Complex to Real-Imag : ComplexToRealImag
  Demux : Demux  Outputs=2
  Demux1 : Demux  Outputs=2
  Gain : Gain  Gain=2*F
  Gain1 : Gain  Gain=2*F
  Gain2 : Gain  Gain=G
  Integrator : Integrator
  Integrator with Wrapped State (Discrete or Continuous) : eeGeneralControl/Integrator with Wrapped State (Discrete or Continuous)  LabelModeActiveChoice=Continuous  WrappedStateUpperValue=2*pi  WrappedStateLowerValue=0  x0=0  Ts=0
  Integrator1 : Integrator
  Math Function : Math  Operator=conj  SignedPower=on
  Mux1 : Mux  Inputs=2
  Product1 : Product
  Product2 : Product
  Product3 : Product
  Radial frequencies : Constant  Value=2*pi*F*K
  Real-Imag to Complex : RealImagToComplex
  Real-Imag to Complex1 : RealImagToComplex
  Subtract : Sum  Inputs=+-
  Subtract1 : Sum  Inputs=+-
  To Workspace17 : ToWorkspace  VariableName=PF3  SaveFormat=Timeseries  SampleTime=0.001
  Transport Delay : TransportDelay  DelayTime=1/F  BufferSize=4096
  Transport Delay1 : TransportDelay  DelayTime=1/F  BufferSize=4096
  Trigonometric Function1 : Trigonometry  Operator=sincos
  P : Outport  VectorParamsAs1DForOutWhenUnconnected=off
  Q : Outport  Port=2  VectorParamsAs1DForOutWhenUnconnected=off
  wires:
  Trigonometric Function1/2 -> Mux1/2
  Radial frequencies/1 -> Integrator with Wrapped State (Discrete or Continuous)/1
  Integrator/1 -> Subtract/1, Transport Delay/1
  Transport Delay/1 -> Subtract/2
  Subtract/1 -> Gain/1
  i/1 -> Product2/1
  Math Function/1 -> Product3/2
  Product3/1 -> Gain2/1
  Real-Imag to Complex/1 -> Product3/1
  Complex to Real-Imag/1 -> Atan2/2, P/1
  Complex to Real-Imag/2 -> Atan2/1, Q/1
  Integrator with Wrapped State (Discrete or Continuous)/1 -> Trigonometric Function1/1
  Real-Imag to Complex1/1 -> Math Function/1
  Gain2/1 -> Complex to Real-Imag/1
  Demux/1 -> Real-Imag to Complex/1
  Gain/1 -> Demux/1
  Demux/2 -> Real-Imag to Complex/2
  Trigonometric Function1/1 -> Mux1/1
  Product1/1 -> Integrator/1
  v/1 -> Product1/1
  Mux1/1 -> Product2/2, Product1/2
  Product2/1 -> Integrator1/1
  Demux1/2 -> Real-Imag to Complex1/2
  Gain1/1 -> Demux1/1
  Demux1/1 -> Real-Imag to Complex1/1
  Subtract1/1 -> Gain1/1
  Transport Delay1/1 -> Subtract1/2
  Integrator1/1 -> Transport Delay1/1, Subtract1/1
  Atan2/1 -> Atan1/1
  Atan1/1 -> To Workspace17/1

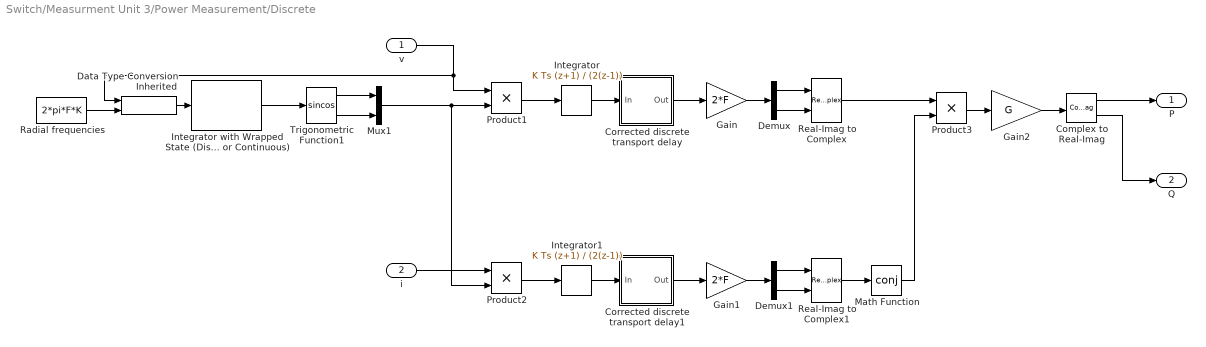
== system Switch/Measurment Unit 3/Power Measurement/Discrete ==
  v : Inport
  i : Inport  Port=2
  Complex to Real-Imag : ComplexToRealImag
  Corrected discrete transport delay : Subsystem
  Corrected discrete transport delay1 : Subsystem
  Data Type Conversion Inherited : simulink/Signal Attributes/Data Type Conversion Inherited  ConvertRealWorld=Real World Value  DoSatur=off
  Demux : Demux  Outputs=2
  Demux1 : Demux  Outputs=2
  Gain : Gain  Gain=2*F
  Gain1 : Gain  Gain=2*F
  Gain2 : Gain  Gain=G
  Integrator : DiscreteIntegrator  IntegratorMethod=Integration: Trapezoidal  SampleTime=Ts  ICPrevOutput=DiscIntNeverNeededParam  ICPrevScaledInput=DiscIntNeverNeededParam  mask(DiscretizedDiscreteIntegrator){}
      mask init:
      | %zoh
  Integrator with Wrapped State (Discrete or Continuous) : eeGeneralControl/Integrator with Wrapped State (Discrete or Continuous)  LabelModeActiveChoice=Continuous  WrappedStateUpperValue=2*pi  WrappedStateLowerValue=0  x0=0  Ts=Ts
  Integrator1 : DiscreteIntegrator  IntegratorMethod=Integration: Trapezoidal  SampleTime=Ts  ICPrevOutput=DiscIntNeverNeededParam  ICPrevScaledInput=DiscIntNeverNeededParam  mask(DiscretizedDiscreteIntegrator){}
      mask init:
      | %zoh
  Math Function : Math  Operator=conj  SignedPower=on
  Mux1 : Mux  Inputs=2
  Product1 : Product
  Product2 : Product
  Product3 : Product
  Radial frequencies : Constant  Value=2*pi*F*K
  Real-Imag to Complex : RealImagToComplex
  Real-Imag to Complex1 : RealImagToComplex
  Trigonometric Function1 : Trigonometry  Operator=sincos
  P : Outport  VectorParamsAs1DForOutWhenUnconnected=off
  Q : Outport  Port=2  VectorParamsAs1DForOutWhenUnconnected=off
  wires:
  Radial frequencies/1 -> Data Type Conversion Inherited/2
  Data Type Conversion Inherited/1 -> Integrator with Wrapped State (Discrete or Continuous)/1
  Trigonometric Function1/2 -> Mux1/2
  Mux1/1 -> Product2/2, Product1/2
  Integrator/1 -> Corrected discrete transport delay/1(In)
  Gain2/1 -> Complex to Real-Imag/1
  Demux1/1 -> Real-Imag to Complex1/1
  Product3/1 -> Gain2/1
  Product1/1 -> Integrator/1
  Gain1/1 -> Demux1/1
  v/1 -> Product1/1, Data Type Conversion Inherited/1
  Integrator1/1 -> Corrected discrete transport delay1/1(In)
  i/1 -> Product2/1
  Complex to Real-Imag/2 -> Q/1
  Gain/1 -> Demux/1
  Trigonometric Function1/1 -> Mux1/1
  Corrected discrete transport delay/1(Out) -> Gain/1
  Math Function/1 -> Product3/2
  Integrator with Wrapped State (Discrete or Continuous)/1 -> Trigonometric Function1/1
  Demux/2 -> Real-Imag to Complex/2
  Corrected discrete transport delay1/1(Out) -> Gain1/1
  Real-Imag to Complex1/1 -> Math Function/1
  Complex to Real-Imag/1 -> P/1
  Real-Imag to Complex/1 -> Product3/1
  Demux1/2 -> Real-Imag to Complex1/2
  Demux/1 -> Real-Imag to Complex/1
  Product2/1 -> Integrator1/1

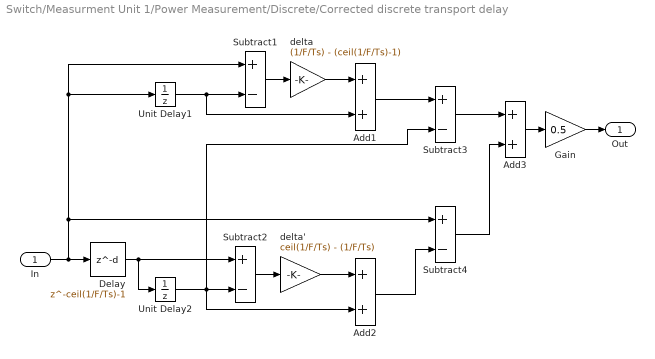
== system Switch/Measurment Unit 1/Power Measurement/Discrete/Corrected discrete transport delay ==
  In : Inport
  Add1 : Sum
  Add2 : Sum
  Add3 : Sum
  Delay : Delay  DelayLength=ceil(1/F/Ts)-1
  Gain : Gain  Gain=0.5
  Subtract{1..4} (4 alike) : Sum  Inputs=+-
  Unit Delay1 : UnitDelay  SampleTime=Ts  HasFrameUpgradeWarning=on
  Unit Delay2 : UnitDelay  SampleTime=Ts  HasFrameUpgradeWarning=on
  delta : Gain  Gain=(1/F/Ts) - (ceil(1/F/Ts)-1)
  delta' : Gain  Gain=ceil(1/F/Ts) - (1/F/Ts)
  Out : Outport  VectorParamsAs1DForOutWhenUnconnected=off
  wires:
  Gain/1 -> Out/1
  Add3/1 -> Gain/1
  Add1/1 -> Subtract3/1
  Unit Delay2/1 -> Subtract2/2, Add2/2, Subtract3/2
  delta/1 -> Add1/1
  delta'/1 -> Add2/1
  Subtract2/1 -> delta'/1
  Subtract4/1 -> Add3/2
  In/1 -> Subtract1/1, Unit Delay1/1, Subtract4/1, Delay/1
  Unit Delay1/1 -> Add1/2, Subtract1/2
  Delay/1 -> Unit Delay2/1, Subtract2/1
  Subtract3/1 -> Add3/1
  Subtract1/1 -> delta/1
  Add2/1 -> Subtract4/2

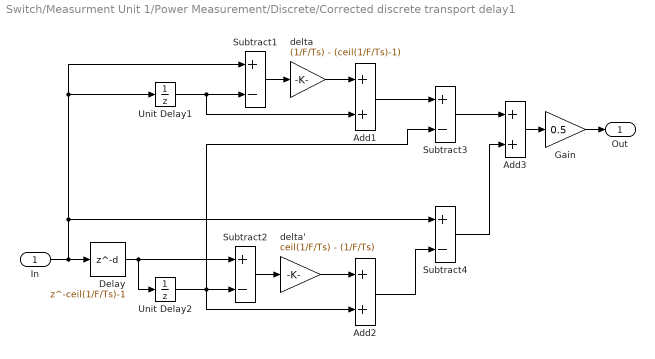
== system Switch/Measurment Unit 1/Power Measurement/Discrete/Corrected discrete transport delay1 ==
  In : Inport
  Add1 : Sum
  Add2 : Sum
  Add3 : Sum
  Delay : Delay  DelayLength=ceil(1/F/Ts)-1
  Gain : Gain  Gain=0.5
  Subtract{1..4} (4 alike) : Sum  Inputs=+-
  Unit Delay1 : UnitDelay  SampleTime=Ts  HasFrameUpgradeWarning=on
  Unit Delay2 : UnitDelay  SampleTime=Ts  HasFrameUpgradeWarning=on
  delta : Gain  Gain=(1/F/Ts) - (ceil(1/F/Ts)-1)
  delta' : Gain  Gain=ceil(1/F/Ts) - (1/F/Ts)
  Out : Outport  VectorParamsAs1DForOutWhenUnconnected=off
  wires:
  Add2/1 -> Subtract4/2
  Subtract1/1 -> delta/1
  Subtract3/1 -> Add3/1
  Delay/1 -> Subtract2/1, Unit Delay2/1
  Unit Delay1/1 -> Subtract1/2, Add1/2
  In/1 -> Delay/1, Subtract4/1, Unit Delay1/1, Subtract1/1
  Subtract4/1 -> Add3/2
  Subtract2/1 -> delta'/1
  delta'/1 -> Add2/1
  delta/1 -> Add1/1
  Unit Delay2/1 -> Subtract3/2, Add2/2, Subtract2/2
  Add1/1 -> Subtract3/1
  Add3/1 -> Gain/1
  Gain/1 -> Out/1

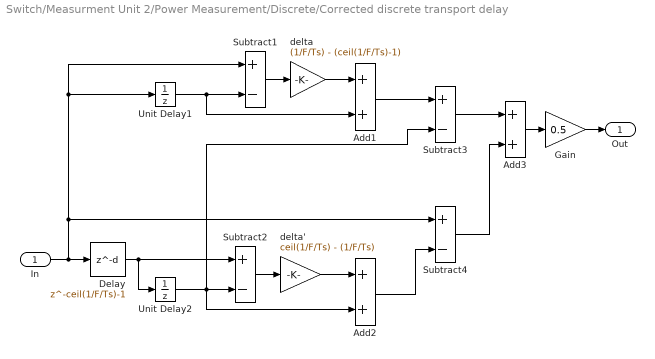
== system Switch/Measurment Unit 2/Power Measurement/Discrete/Corrected discrete transport delay ==
  In : Inport
  Add1 : Sum
  Add2 : Sum
  Add3 : Sum
  Delay : Delay  DelayLength=ceil(1/F/Ts)-1
  Gain : Gain  Gain=0.5
  Subtract{1..4} (4 alike) : Sum  Inputs=+-
  Unit Delay1 : UnitDelay  SampleTime=Ts  HasFrameUpgradeWarning=on
  Unit Delay2 : UnitDelay  SampleTime=Ts  HasFrameUpgradeWarning=on
  delta : Gain  Gain=(1/F/Ts) - (ceil(1/F/Ts)-1)
  delta' : Gain  Gain=ceil(1/F/Ts) - (1/F/Ts)
  Out : Outport  VectorParamsAs1DForOutWhenUnconnected=off
  wires:
  Add2/1 -> Subtract4/2
  Subtract1/1 -> delta/1
  Subtract3/1 -> Add3/1
  Delay/1 -> Subtract2/1, Unit Delay2/1
  Unit Delay1/1 -> Subtract1/2, Add1/2
  In/1 -> Delay/1, Subtract4/1, Unit Delay1/1, Subtract1/1
  Subtract4/1 -> Add3/2
  Subtract2/1 -> delta'/1
  delta'/1 -> Add2/1
  delta/1 -> Add1/1
  Unit Delay2/1 -> Subtract3/2, Add2/2, Subtract2/2
  Add1/1 -> Subtract3/1
  Add3/1 -> Gain/1
  Gain/1 -> Out/1

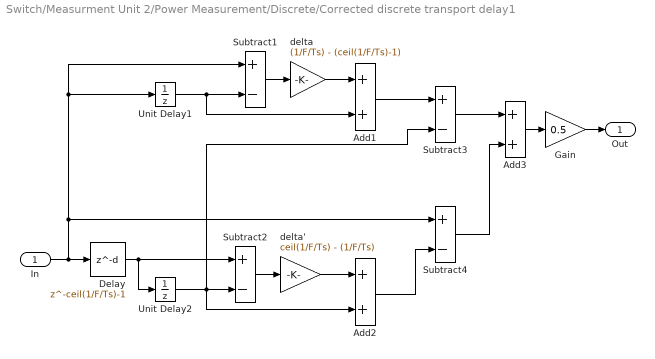
== system Switch/Measurment Unit 2/Power Measurement/Discrete/Corrected discrete transport delay1 ==
  In : Inport
  Add1 : Sum
  Add2 : Sum
  Add3 : Sum
  Delay : Delay  DelayLength=ceil(1/F/Ts)-1
  Gain : Gain  Gain=0.5
  Subtract{1..4} (4 alike) : Sum  Inputs=+-
  Unit Delay1 : UnitDelay  SampleTime=Ts  HasFrameUpgradeWarning=on
  Unit Delay2 : UnitDelay  SampleTime=Ts  HasFrameUpgradeWarning=on
  delta : Gain  Gain=(1/F/Ts) - (ceil(1/F/Ts)-1)
  delta' : Gain  Gain=ceil(1/F/Ts) - (1/F/Ts)
  Out : Outport  VectorParamsAs1DForOutWhenUnconnected=off
  wires:
  Gain/1 -> Out/1
  Add3/1 -> Gain/1
  Add1/1 -> Subtract3/1
  Unit Delay2/1 -> Subtract2/2, Add2/2, Subtract3/2
  delta/1 -> Add1/1
  delta'/1 -> Add2/1
  Subtract2/1 -> delta'/1
  Subtract4/1 -> Add3/2
  In/1 -> Subtract1/1, Unit Delay1/1, Subtract4/1, Delay/1
  Unit Delay1/1 -> Add1/2, Subtract1/2
  Delay/1 -> Unit Delay2/1, Subtract2/1
  Subtract3/1 -> Add3/1
  Subtract1/1 -> delta/1
  Add2/1 -> Subtract4/2

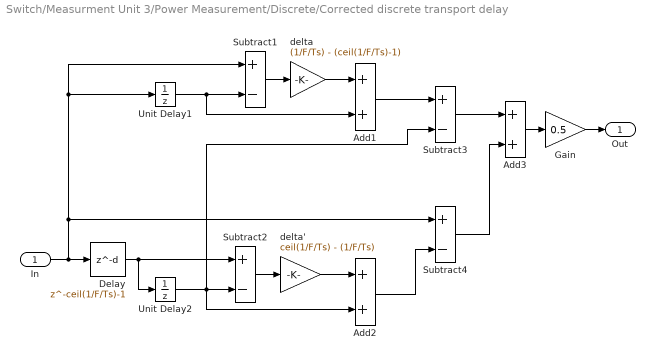
== system Switch/Measurment Unit 3/Power Measurement/Discrete/Corrected discrete transport delay ==
  In : Inport
  Add1 : Sum
  Add2 : Sum
  Add3 : Sum
  Delay : Delay  DelayLength=ceil(1/F/Ts)-1
  Gain : Gain  Gain=0.5
  Subtract{1..4} (4 alike) : Sum  Inputs=+-
  Unit Delay1 : UnitDelay  SampleTime=Ts  HasFrameUpgradeWarning=on
  Unit Delay2 : UnitDelay  SampleTime=Ts  HasFrameUpgradeWarning=on
  delta : Gain  Gain=(1/F/Ts) - (ceil(1/F/Ts)-1)
  delta' : Gain  Gain=ceil(1/F/Ts) - (1/F/Ts)
  Out : Outport  VectorParamsAs1DForOutWhenUnconnected=off
  wires:
  Add2/1 -> Subtract4/2
  Subtract1/1 -> delta/1
  Subtract3/1 -> Add3/1
  Delay/1 -> Subtract2/1, Unit Delay2/1
  Unit Delay1/1 -> Subtract1/2, Add1/2
  In/1 -> Delay/1, Subtract4/1, Unit Delay1/1, Subtract1/1
  Subtract4/1 -> Add3/2
  Subtract2/1 -> delta'/1
  delta'/1 -> Add2/1
  delta/1 -> Add1/1
  Unit Delay2/1 -> Subtract3/2, Add2/2, Subtract2/2
  Add1/1 -> Subtract3/1
  Add3/1 -> Gain/1
  Gain/1 -> Out/1

== system Switch/Measurment Unit 3/Power Measurement/Discrete/Corrected discrete transport delay1 ==
  In : Inport
  Add1 : Sum
  Add2 : Sum
  Add3 : Sum
  Delay : Delay  DelayLength=ceil(1/F/Ts)-1
  Gain : Gain  Gain=0.5
  Subtract{1..4} (4 alike) : Sum  Inputs=+-
  Unit Delay1 : UnitDelay  SampleTime=Ts  HasFrameUpgradeWarning=on
  Unit Delay2 : UnitDelay  SampleTime=Ts  HasFrameUpgradeWarning=on
  delta : Gain  Gain=(1/F/Ts) - (ceil(1/F/Ts)-1)
  delta' : Gain  Gain=ceil(1/F/Ts) - (1/F/Ts)
  Out : Outport  VectorParamsAs1DForOutWhenUnconnected=off
  wires:
  Gain/1 -> Out/1
  Add3/1 -> Gain/1
  Add1/1 -> Subtract3/1
  Unit Delay2/1 -> Subtract2/2, Add2/2, Subtract3/2
  delta/1 -> Add1/1
  delta'/1 -> Add2/1
  Subtract2/1 -> delta'/1
  Subtract4/1 -> Add3/2
  In/1 -> Subtract1/1, Unit Delay1/1, Subtract4/1, Delay/1
  Unit Delay1/1 -> Add1/2, Subtract1/2
  Delay/1 -> Unit Delay2/1, Subtract2/1
  Subtract3/1 -> Add3/1
  Subtract1/1 -> delta/1
  Add2/1 -> Subtract4/2
